simulink model "TV_2017old"  (R2016a)
settings: Solver=FixedStepAuto  StartTime=0.0  StopTime=inf  FixedStep=0.001  RelTol=1e-3
PreLoadFcn:
  | TV_2017_parameters
values from neighbouring files (symbols this model uses):
  battery_voltage = single(530)    [HIL_parameters.m]    (also in HIL_parameters_2018.m; TV_2017_parameters.m; TV_2017_parameters_VD.m)
  car_params = Simulink_Car_params    [HIL_parameters.m]    (also in HIL_parameters_2018.m; TV_2017_parameters.m; TV_2017_parameters_VD.m)
  i_Diff = 16    [HIL_parameters.m]    (also in HIL_parameters_2018.m; TV_2017_parameters.m)
  Kp = 1    [HIL_parameters.m]    (also in HIL_parameters_2018.m; TV_2017_parameters.m; TV_2017_parameters_VD.m)
  motor_data = struct    [HIL_parameters.m]    (also in HIL_parameters_2018.m; TV_2017_parameters.m)
  powerLimitControl = Simulink_el    [HIL_parameters.m]    (also in HIL_parameters_2018.m; TV_2017_parameters.m; TV_2017_parameters_VD.m)
  settings = Simulink_Settings    [HIL_parameters.m]    (also in HIL_parameters_2018.m; TV_2017_parameters.m; TV_2017_parameters_VD.m)
  SpdC_BCC = 0    [HIL_parameters.m]    (also in HIL_parameters_2018.m; TV_2017_parameters.m; TV_2017_parameters_VD.m)
  Speed_Neg_sat = -21    [HIL_parameters.m]    (also in HIL_parameters_2018.m; TV_2017_parameters.m; TV_2017_parameters_VD.m)
  Speed_Pos_sat = 21    [HIL_parameters.m]    (also in HIL_parameters_2018.m; TV_2017_parameters.m; TV_2017_parameters_VD.m)
  SteeringAngleFL = [-23.80 -22.65 -21.50 -20.34 -19.18 -18.03 -16.86 -15.70 -14.53 -13.35 -12.18 -10.99 -9.80 -8.61 -7.40 -6.19 -4.97 -3.75 -2.51 -1.26 0 1.27 2.56 3.85 5.17 6.50 7.84 9.21 10.59 12.00 13.42 14.88 16.36 17.87 19.41 20.99 22.61 24.26 25.97 27.73 29.54]    [CarSetupAnalysis2018.m]    (also in HIL_parameters_2018.m; TV_2017_parameters.m; TV_2017_parameters_VD.m = [-24.129 -22.950 -21.772 -20.593 -19.413 -18.232 -17.050 -15)
  SteeringAngleFR = [-29.54 -27.73 -25.97 -24.26 -22.61 -20.99 -19.41 -17.87 -16.36 -14.88 -13.42 -12.00 -10.59 -9.21 -7.84 -6.50 -5.17 -3.85 -2.56 -1.27 0 1.26 2.51 3.75 4.97 6.19 7.40 8.61 9.80 10.99 12.18 13.35 14.53 15.70 16.86 18.03 19.18 20.34 21.50 22.65 23.80]    [CarSetupAnalysis2018.m]    (also in HIL_parameters_2018.m; TV_2017_parameters.m; TV_2017_parameters_VD.m = [-29.3050 -27.5340 -25.8140 -24.1410 -22.5110 -20.9180 -19.3)
  SteeringWhAngle = [-105 -99.75 -94.5 -89.25 -84 -78.75 -73.5 -68.25 -63 -57.75 -52.5 -47.25 -42 -36.75 -31.5 -26.25 -21.0 -15.75 -10.5 -5.25 0.0 5.25 10.50 15.75 21.00 26.25 31.50 36.75 42.00 47.25 52.50 57.75  63.00 68.25 73.50 78.75 84.00 89.25 94.50 99.75 105.00]    [TV_2017_parameters_VD.m]
  Tn_n = 0    [HIL_parameters.m]    (also in HIL_parameters_2018.m; TV_2017_parameters.m; TV_2017_parameters_VD.m)
  tractionControl = Simulink_tc    [HIL_parameters.m]    (also in HIL_parameters_2018.m; IterativeTractionControlTuning.m; TV_2017_parameters.m; TV_2017_parameters_VD.m)
  yawRateControl = Simulink_yawRate    [HIL_parameters.m]    (also in HIL_parameters_2018.m; TV_2017_parameters.m; TV_2017_parameters_VD.m)
undefined symbols (not defined in the file or in its folder): DiscIntNeverNeededParam, magnitude, speedEstimation, TC_Decr_Gas, TC_Derivative, TC_Incr_Gas, TC_On, TC_Relay_Off, TC_Relay_On
libraries: CarMaker4SL x274, simulink_extras x45, simulink x37, dspfdesign x2
(part 8 of 14)

== matlab function TV_2017old/CarMaker/Estimations/EstimateVx/velocity_Estimation ==
  data: sensors input Bus: SensorInputs; V_est_x output; normalForces input Bus: normalForces; settings parameter; car_params parameter; speedEstimation parameter
function V_est_x  = velocityEstimation(sensors,normalForces,settings,car_params,speedEstimation)
%#codegen


persistent firstIteration;
persistent v;
persistent error;
persistent K;
persistent drift;

k_FL = single(0); % Gain 
k_FR = single(0); % Gain
k_RL = single(0); % Gain
k_RR = single(0); % Gain
% Gains for trusting, not trusting wheel speed measurements
Hg = speedEstimation.High_gain;
Lg = speedEstimation.Low_gain;
% Variances
all_Var = single(0); % Variance for all measurements
front_rear_Var = single(0);
front_Var = single(0);
rear_Var = single(0);
left_Var = single(0);
right_Var = single(0);
% LIMITS:
velocity_deviation_limit = speedEstimation.velocity_deviation_limit;
lim = speedEstimation.variance_limit;
RPM_derivative_limit = speedEstimation.RPM_derivative_limit;

% Measurement vector
C = [1;1;1;1]; % Create four copies of predicted vx


c = single(2*pi/(car_params.GR*60));

t = settings.control_system_sample_time;
%Weights taken from wikipedia
%sg_Weight = single( [ 1; -8; 0; 8; -1] );
sg_Weight = single( [ -1; 8; 0; -8; 1] );
%sg_Weight = single([0.3; 0.1; -0.1 ; -0.3]);
%sg_Weight = single([1; -1; 0 ; -0]);
% ------------------------------
% COPY VARIABLES EACH TIMESTEP
% ------------------------------
S = sensors.steering_wheel_angle; % Steering angle in rad( Mean of front wheels)
ax = sensors.ax; % Should be true linear acceleration compensated for roll angle
%Fz, used to determine what wheel speeds to trust.
Fz = [normalForces.FL, normalForces.FR, normalForces.RL ,normalForces.RR];
% Determine CoG Vx from motor RPM. Simple atm. Not considering vy.
Whl_v_FL = sensors.RPM_FL*c*car_params.r_eff*cos(S) + sensors.yawRate*car_params.t_f;
Whl_v_FR = sensors.RPM_FR*c*car_params.r_eff*cos(S) - sensors.yawRate*car_params.t_f;
Whl_v_RL = sensors.RPM_RL*c*car_params.r_eff + sensors.yawRate*car_params.t_r;
Whl_v_RR = sensors.RPM_RR*c*car_params.r_eff - sensors.yawRate*car_params.t_r;
whl_speed.v_FL = Whl_v_FL;
whl_speed.v_FR = Whl_v_FR;
whl_speed.v_RL = Whl_v_RL;
whl_speed.v_RR = Whl_v_RR;


RPM = [sensors.RPM_FL, sensors.RPM_FR, sensors.RPM_RL, sensors.RPM_RR]';
% Measurement vector, compensated RPMS
Y_meas = [Whl_v_FL, Whl_v_FR, Whl_v_RL, Whl_v_RR]';
% Input Derivative of RPM
rateRPM_FL = sensors.RPM_der_FL;
rateRPM_FR = sensors.RPM_der_FR;
rateRPM_RL = sensors.RPM_der_RL;
rateRPM_RR = sensors.RPM_der_RR;

% Different sums of normal forces, used to determine what wheels to trust
left_Fz = sum(Fz([1 3]));
right_Fz = sum(Fz([2 4]));
front_Fz = sum(Fz(1:2));
rear_Fz = sum(Fz(3:4));
% ALGORITHM
if (isempty(firstIteration))
    K = single(ones(1,4));
    v = single(0);
    V_est_x = v;
    error = Y_meas- C*v;
    firstIteration = 2;
    drift = single(0);
else
    v_ins = sensors.V_x_INS + 0.05 + drift;
    mean_WhlV = max(0.001,mean(Y_meas));
    mean_front_WhlV = max(0.001,mean(Y_meas(1:2)));
    mean_rear_WhlV  = max(0.001,mean(Y_meas(3:4)));
    mean_left_WhlV  = max(0.001,mean(Y_meas([1 3])));
    mean_right_WhlV = max(0.001,mean(Y_meas([2 4])));

    all_Var = var(Y_meas,1)/mean_WhlV;
    front_rear_Var = var([mean_front_WhlV, mean_rear_WhlV],1)/mean_WhlV;
    front_Var = var(Y_meas(1:2),1)/mean_front_WhlV;
    rear_Var  = var(Y_meas(3:4),1)/mean_rear_WhlV;
    
    left_Var    = var(Y_meas([1 3]),1)/mean_left_WhlV;
    right_Var   = var(Y_meas([2 4]),1)/mean_right_WhlV;   
    
    if ( (abs(Whl_v_FL - v_ins) > velocity_deviation_limit)...
       && (abs(Whl_v_FR - v_ins) > velocity_deviation_limit)...
       && (abs(Whl_v_RL - v_ins) > velocity_deviation_limit)...
       && (abs(Whl_v_RR - v_ins) > velocity_deviation_limit) )
        
        K = [Lg, Lg, Lg, Lg];
    elseif (all_Var  < lim ) 
        % low variance for all wheels.
        % Check derivative of motor RPM
        if ( (rateRPM_FL > RPM_derivative_limit) ||...
             (rateRPM_FR > RPM_derivative_limit) ||...
             (rateRPM_RL > RPM_derivative_limit) ||...
             (rateRPM_RR > RPM_derivative_limit))
            K = [Lg, Lg, Lg, Lg];
        % Rate of change of RPM can be low but slip rate is large
        % Check against drifting INS velocity 
        else
            K = [Hg, Hg ,Hg ,Hg];
        end
    % Variance is high. What wheel(s) are causing this.. 
    % STRUCTURE:
    % 1 = FRONT AND REAR DIFFER
    % 2 = LEFT AND RIGHT DIFFER
    % 3 = FL WRONG
    % 4 = FR WRONG
    % 5 = RL WRONG
    % 6 = RR WRONG
    % 7 Combinations of 3-6 that are not handled in 1-2.
    
    %1: FRONT AND REAR DIFFER
    elseif( (right_Var > front_Var) && (right_Var > rear_Var)...
            && (left_Var > front_Var) && (left_Var > rear_Var))
        % High variance between front and rear, and low variance 
        % at front and rear.
        
        % Also need to check if front/rear wheels are slippin    
        % Front wheels over limit while rear is ok
        if (((rateRPM_FL > RPM_derivative_limit) ||...
             (rateRPM_FR > RPM_derivative_limit)) &&...
            ((rateRPM_RL < RPM_derivative_limit) ||...
             (rateRPM_RR < RPM_derivative_limit)) )
             
            K = [Lg, Lg, Hg, Hg];
        % Rear wheels over limit while front is ok
        elseif ( ((rateRPM_FL < RPM_derivative_limit) ||...
                 (rateRPM_FR < RPM_derivative_limit)) &&...
                ((rateRPM_RL > RPM_derivative_limit) ||...
                 (rateRPM_RR > RPM_derivative_limit)) )
             K = [Hg, Hg, Lg, Lg];
        % All are over limit
        elseif  ((rateRPM_FL > RPM_derivative_limit) &&...
                 (rateRPM_FR > RPM_derivative_limit) &&...
                 (rateRPM_RL > RPM_derivative_limit) &&...
                 (rateRPM_RR > RPM_derivative_limit) ) 
              K = [Lg, Lg, Lg, Lg];
              
        % The rate of change of RPM will flatten out and the high
        % slip ratio will still exist. Handle this
        
        % Check big difference in wheel speeds
        % Two cases. Driving and braking. 
        
        % Driving. Need logic to determine driving/braking
        elseif ( (RPM(1) + RPM(2)) > (RPM(3) + RPM(4)) )
            K = [Lg, Lg, Hg, Hg];
        elseif ( (RPM(1) + RPM(2)) < (RPM(3) + RPM(4)) )
            K = [Hg, Hg, Lg, Lg];
            % If frontFZ - rearFZ < 0, then FL is set to 0
            % Else it is set to a positive gain
%             k_FL = (1/abs(front_Fz-rear_Fz))*max(0,front_Fz - rear_Fz);
%             k_FR = (1/abs(front_Fz-rear_Fz))*max(0,front_Fz - rear_Fz);
% 
%             k_RL = (1/abs(rear_Fz-front_Fz))*max(0,rear_Fz-front_Fz)*0.5;
%             k_RR = (1/abs(rear_Fz-front_Fz))*max(0,rear_Fz-front_Fz)*0.5;
%            K = [k_FL, k_FR, k_RL, k_RR];
        end
    %2: LEFT AND RIGHT WHEELS DIFFER
    elseif ( ((front_Var > right_Var) && (rear_Var > right_Var)) ||...
            ( (front_Var > left_Var) && (rear_Var > left_Var)))
   
        k_FL = (1/abs(left_Fz-right_Fz))*max(0,left_Fz - right_Fz);
        k_RL = (1/abs(left_Fz-right_Fz))*max(0,left_Fz - right_Fz);
        
        k_FR = (1/abs(right_Fz-left_Fz))*max(0,right_Fz-left_Fz);
        k_RR = (1/abs(right_Fz-left_Fz))*max(0,right_Fz-left_Fz);
        
        K = [k_FL, k_FR, k_RL, k_RR];
        
    %3: FL WRONG
    elseif ( (left_Var > rear_Var) && (left_Var > right_Var)...
            && (front_Var > rear_Var) )
        k_FL = single(0);
        k_FR = single(0);
        k_RL = single(1);
        k_RR = single(1);
        K = [k_FL, k_FR, k_RL, k_RR];
    %4: FR WRONG
    elseif ( (right_Var > rear_Var) && (right_Var > left_Var)...
            && (front_Var > rear_Var))
        k_FL = single(0);
        k_FR = single(0);
        k_RL = single(1);
        k_RR = single(1);
        K = [k_FL, k_FR, k_RL, k_RR]; 
    %5: RL WRONG
    elseif ( (left_Var > front_Var) && (left_Var > right_Var)...
            && (rear_Var > front_Var))
        
        k_FL = single(1);
        k_FR = single(1);
        k_RL = single(0);
        k_RR = single(0);
        K = [k_FL, k_FR, k_RL, k_RR]; 
        
    %5: RR WRONG    
    elseif ( (right_Var > front_Var) && (right_Var > left_Var)...
            && (rear_Var > front_Var))
        k_FL = single(1);
        k_FR = single(1);
        k_RL = single(0);
        k_RR = single(0);
        K = [k_FL, k_FR, k_RL, k_RR]; 
    else
        k_FL = single(0);
        k_FR = single(0);
        k_RL = single(0);
        k_RR = single(0);
        K = [k_FL, k_FR, k_RL, k_RR]; 
    end
    
    drift = drift + 0.03*t;
   
    %v = v + t*ax;
    v = v + t*(ax + K*error);
    error = Y_meas - C*v ;
    V_est_x = 0.98*v;
end
end

== matlab function TV_2017old/CarMaker/Control_System /Throttle // Brake Mapping ==
  data: states input; settings parameter; T_req output; car_params parameter
function T_req = pedalMapping(states,settings,car_params)
%#codegen

    KERS_pos = states.KERS_pos;
    throttle = min(1,states.Input_throttle);
    T_req = single(0);
    Fx_req = single(0);
    max_drive_torque = settings.max_motor_torque*4;
    max_brake_torque = settings.max_motor_brake_torque*4;
    
   persistent firstIteration;
   persistent KERS_allowed;
   
   % Hysteresis on KERS pedal input to avoid oscillation around 
   % allowed KERS speed. 
   if isempty(firstIteration)
      firstIteration = 2; %
      KERS_allowed = uint32(0);
   else
      % Hysteresis around the minimum KERS speed
       if     ( (KERS_allowed == 0) && (states.V_x > settings.KERS_speed_limit_hyst_high) )
           KERS_allowed = uint32(1);
       elseif ( (KERS_allowed == 1) && (states.V_x < settings.KERS_speed_limit_hyst_low) )
           KERS_allowed = uint32(0);
       end          
   end   
  if (settings.KERS_active == 1) 
      T_req = max_drive_torque*throttle  -  max_brake_torque*KERS_pos * single(KERS_allowed) ;
  else
      T_req = max_drive_torque*throttle ;
  end  
end

== matlab function TV_2017old/CarMaker/Estimations/Fz_Estimation_acceleration based/Fz_acc_est ==
  data: sensors input Bus: SensorInputs; Fz_acc_est output Bus: normalForces; car_params parameter; alfa_r_acc output
function [Fz_acc_est, alfa_r_acc] =  FzEstAcc(sensors , car_params)
%#codegen
g = 9.81;
ax = sensors.ax;
ay = sensors.ay;

total_mass = 245;
sprung_mass = 124+70;
unsprung_front = car_params.unsprung_mass_per_wheel_newton_front;
unspring_rear = car_params.unsprung_mass_per_wheel_newton_rear;
cg_z = 0.300;%car_params.CoG_height;
t_f = car_params.t_f;
t_r = car_params.t_r;
l_f = car_params.l_f;%Distance CoG to front axle
l_r = car_params.l_r;%Distance CoG to rear axle

K_ax = 1.25;
K_ay = 1.20;

%estimate forces from spring, damper and ARB
Fz_acc_est.FL = g*sprung_mass*0.25 + unsprung_front - K_ax*0.25*ax*sprung_mass*cg_z/l_f - K_ay*0.25*ay*sprung_mass*cg_z/t_f;
Fz_acc_est.FR = g*sprung_mass*0.25 + unsprung_front - K_ax*0.25*ax*sprung_mass*cg_z/l_f + K_ay*0.25*ay*sprung_mass*cg_z/t_f;
Fz_acc_est.RL = g*sprung_mass*0.25 + unspring_rear  + K_ax*0.25*ax*sprung_mass*cg_z/l_r - K_ay*0.25*ay*sprung_mass*cg_z/t_r;
Fz_acc_est.RR = g*sprung_mass*0.25 + unspring_rear  + K_ax*0.25*ax*sprung_mass*cg_z/l_r + K_ay*0.25*ay*sprung_mass*cg_z/t_r;

alfa_r_acc = (1.5+ax/g)/(3);

== matlab function TV_2017old/CarMaker/Estimations/SR_Calculation/Slip ratio ==
  data: V_x input; SR output Bus: SR; whl_v input Bus: Whl_speed; sensor input; car_params parameter
function SR = slipRatioCalculation(V_x,whl_v,sensor,car_params)
%#codegen

vx_to_wheel_factor = single(0.6);
vx_omega = sensor.yawRate*vx_to_wheel_factor;

Vx_FL = -vx_omega + V_x;
Vx_FR =  vx_omega + V_x;
Vx_RL = -vx_omega + V_x;
Vx_RR =  vx_omega + V_x;


SR.FL = single((whl_v.FL - Vx_FL) / max([1, abs(Vx_FL)]));    
SR.FR = single((whl_v.FR - Vx_FR) / max([1, abs(Vx_FR)]));
SR.RL = single((whl_v.RL - Vx_RL) / max([1, abs(Vx_RL)]));
SR.RR = single((whl_v.RR - Vx_RR) / max([1, abs(Vx_RR)]));

end

== matlab function TV_2017old/CarMaker/Estimations/RPM_to_linearVelocity/whl_v_calculation ==
  data: sensors input Bus: SensorInputs; meanWheelAngle input; car_params parameter; whl_speed output Bus: Whl_speed
function whl_speed = rpmToWhlVelocity(sensors,meanWheelAngle,car_params)
%#codegen

S = meanWheelAngle; % Steering angle in rad( Mean of front wheels)
c = single(2*pi/(car_params.GR*60));

% Determine CoG Vx from motor RPM. Simple atm. Not considering vy.
whl_speed.FL = sensors.RPM_FL*c*car_params.r_eff*cos(S) ;%+ sensors.yawRate*car_params.t_f;
whl_speed.FR = sensors.RPM_FR*c*car_params.r_eff*cos(S) ;%- sensors.yawRate*car_params.t_f;
whl_speed.RL = sensors.RPM_RL*c*car_params.r_eff        ;%+ sensors.yawRate*car_params.t_r;
whl_speed.RR = sensors.RPM_RR*c*car_params.r_eff        ;%- sensors.yawRate*car_params.t_r;

== matlab function TV_2017old/CarMaker/Estimations/Fx_Estimation/EstimateFx ==
  data: car_params parameter; Fx output Bus: Fx; sensors input Bus: SensorInputs; T_motor output Bus: T_motor
function [Fx, T_motor] = estimateFx(car_params, sensors)
%#codegen
Iq_FL = sensors.Iq_FL;
Iq_FR = sensors.Iq_FR;
Iq_RL = sensors.Iq_RL;
Iq_RR = sensors.Iq_RR;

Id_FL = sensors.Id_FL;
Id_FR = sensors.Id_FR;
Id_RL = sensors.Id_RL;
Id_RR = sensors.Id_RR;

Kt = car_params.Kt;     % Torque constant
Lq = car_params.Lq;     % Quadrature axis inductance 
Ld = car_params.Ld;     % Direct access inductance
Jw = car_params.Jw;     % Motor inertia
R  = car_params.r_eff;  % Radius center of rim to tire contact
GR = car_params.GR;     % Gear ratio
% Convert RPM Derivative to angular acceleration
c = single(2*pi/(GR*60));
ang_acc_FL = c*sensors.RPM_der_FL;
ang_acc_FR = c*sensors.RPM_der_FR;
ang_acc_RL = c*sensors.RPM_der_RL;
ang_acc_RR = c*sensors.RPM_der_RR;

% T_motor.FL = (Iq_FL*Kt*sqrt(2)-(Lq-Ld)*Id_FL);
% T_motor.FR = (Iq_FR*Kt*sqrt(2)-(Lq-Ld)*Id_FR);
% T_motor.RL = (Iq_RL*Kt*sqrt(2)-(Lq-Ld)*Id_RL);
% T_motor.RR = (Iq_RR*Kt*sqrt(2)-(Lq-Ld)*Id_RR);

T_motor.FL = (Iq_FL*Kt);
T_motor.FR = (Iq_FR*Kt);
T_motor.RL = (Iq_RL*Kt);
T_motor.RR = (Iq_RR*Kt);
%T_FL = T_CM.FL;
%T_FR = T_CM.FR;
%T_RL = T_CM.RL;
%T_RR = T_CM.RR;


Fx.FL = (T_motor.FL*GR - Jw*ang_acc_FL)/R;
Fx.FR = (T_motor.FR*GR - Jw*ang_acc_FR)/R;
Fx.RL = (T_motor.RL*GR - Jw*ang_acc_RL)/R;
Fx.RR = (T_motor.RR*GR - Jw*ang_acc_RR)/R;

== matlab function TV_2017old/CarMaker/Estimations/friction_estimation/estimateFrictionCoefficient ==
  data: Fx input Bus: Fx; mu output; mu_estimate output; Fz input Bus: normalForces; SR input Bus: SR; settings parameter; normLongTireForce output Bus: normLongTireForce
function [mu, mu_estimate, normLongTireForce]= estimateFrictionCoefficient(Fx,Fz,SR,settings)
%#codegen
persistent mu_FL;
persistent mu_FR;
persistent mu_RL;
persistent mu_RR;
persistent firstIteration;

mu_forget_factor = 0.001;  %kan legges in som parameter etter hvert. (Emil.17.10.2017)
mu_growth_factor = 0.0001;
mu_shrink_factor = 0.0001;
mu_full_slip_lim = 0.23;
mu_hi_slip_lim   = 0.13;
mu_lo_slip_lim   = 0.09;
mu_no_slip_lim   = 0.05;


if isempty(firstIteration)
    firstIteration = 2; %
    mu_FL = settings.mu;
    mu_FR = settings.mu;
    mu_RL = settings.mu;
    mu_RR = settings.mu;
    normLongTireForce.FL = single(0);
    normLongTireForce.FR = single(0);
    normLongTireForce.RL = single(0);
    normLongTireForce.RR = single(0);
   
      
else
    normLongTireForce.FL = (Fx.FL/Fz.FL);
    normLongTireForce.FR = (Fx.FR/Fz.FR);
    normLongTireForce.RL = (Fx.RL/Fz.RL);
    normLongTireForce.RR = (Fx.RR/Fz.RR);

%     %Front left
%     if (SR.FL > mu_lo_slip_lim) && (SR.FL < mu_hi_slip_lim)
%         mu_FL = (1-mu_forget_factor)*mu_FL + mu_forget_factor*normLongTireForce.FL;
%     elseif (SR.FL > mu_no_slip_lim) && (SR.FL < mu_lo_slip_lim)
%         mu_FL = (1-mu_forget_factor)*mu_FL + mu_growth_factor;
%     elseif (SR.FL > mu_lo_slip_lim) && (SR.FL < mu_full_slip_lim)
%         mu_FL = (1-mu_forget_factor)*mu_FL - mu_shrink_factor;        
%     end
%     %Front right
%     if (SR.FR > mu_lo_slip_lim) && (SR.FR < mu_hi_slip_lim)
%         mu_FR = (1-mu_forget_factor)*mu_FR + mu_forget_factor*normLongTireForce.FR;
%     elseif (SR.FR > mu_no_slip_lim) && (SR.FR < mu_lo_slip_lim)
%         mu_FR = (1-mu_forget_factor)*mu_FR + mu_growth_factor;
%     elseif (SR.FR > mu_lo_slip_lim) && (SR.FR < mu_full_slip_lim)
%         mu_FR = (1-mu_forget_factor)*mu_FR - mu_shrink_factor;        
%     end
%     %Rear left
%     if ( SR.RL > mu_lo_slip_lim) && (SR.RL < mu_hi_slip_lim)
%         mu_RL = (1-mu_forget_factor)*mu_RL + mu_forget_factor*normLongTireForce.RL;
%     elseif (SR.RL > mu_no_slip_lim) && (SR.RL < mu_lo_slip_lim)
%         mu_RL = (1-mu_forget_factor)*mu_RL + mu_growth_factor;
%     elseif (SR.RL > mu_lo_slip_lim) && (SR.RL < mu_full_slip_lim)
%         mu_RL = (1-mu_forget_factor)*mu_RL - mu_shrink_factor;        
%     end
%     %Rear right
%     if (SR.RR > mu_lo_slip_lim) && (SR.RR < mu_hi_slip_lim)
%        mu_RR = (1-mu_forget_factor)*mu_RR + mu_forget_factor*normLongTireForce.RR;
%     elseif (SR.RR > mu_no_slip_lim) && (SR.RR < mu_lo_slip_lim)
%        mu_RR = (1-mu_forget_factor)*mu_RR + mu_growth_factor;
%     elseif (SR.RR > mu_lo_slip_lim) && (SR.RR < mu_full_slip_lim)
%        mu_RR = (1-mu_forget_factor)*mu_RR - mu_shrink_factor;        
%     end
%}
end

mu = settings.mu;
mu_estimate = 0.25*(mu_FL+mu_FR+mu_RL+mu_RR);

end

== matlab function TV_2017old/CarMaker/Estimations/Fz_Estimation/1st_deriv/Diff_Function ==
  data: y_old output; y_old input; sig input; y output; delta_t input
function [y_old,y] = innerFunction(y_old, sig, delta_t)

y_old = circshift(y_old,1);
y_old(1) = sig;
        
M = length(y_old);
N = 3;
nu = 1;
j = 1;

k = 1:M;

x = phi(M,N,nu,j,k,delta_t) .* y_old;

y = sum(x);

end

function p = phi(M,N,nu,j,k,delta_t)

fac = (factorial(N + j + nu + 1) .*...
    factorial(N + 1)) ./...
    (M .* delta_t) .^ j;

[i,k2,k1,k] = ndgrid(0:nu + N,0:j,0:N-j,k);

eliminator = i > nu + k1 + k2;

evalIn = inPhi(M,N,nu,j,k,i,k1,k2);
evalIn(eliminator) = 0;

p = fac * sum(sum(sum(evalIn)));

p = p(:);

end

function p = inPhi(M,N,nu,j,k,i,k1,k2)

p = ((-1).^(N + i - k1 - k2) .*...
    ((k./M).^(N + i - k1 - k2 + 1) - ...
    ((k-1)./M).^(N + i - k1 - k2 + 1)))./...
    (factorial(k1) .* factorial(k2) .* factorial(i).*...
    factorial(N - j - k1) .*...
    factorial(j - k2) .*...
    factorial(N - k1 - k2) .*...
    factorial(nu - i + k1 + k2) .*...
    (N - k1 + 1) .*...
    (N + i -k1 - k2 + 1));

end

function n = factorial(n)

fac = [1;1;2;6;24;120;720;5040;40320;362880;3628800;39916800;479001600;6227020800.00000;87178291200.0000;1307674368000.00;20922789888000.0;355687428096000;6.40237370572800e+15;1.21645100408832e+17;2.43290200817664e+18;5.10909421717094e+19;1.12400072777761e+21;2.58520167388850e+22;6.20448401733239e+23;1.55112100433310e+25;4.03291461126606e+26;1.08888694504184e+28;3.04888344611714e+29;8.84176199373970e+30;2.65252859812191e+32;8.22283865417792e+33;2.63130836933694e+35;8.68331761881189e+36;2.95232799039604e+38;1.03331479663861e+40;3.71993326789901e+41;1.37637530912263e+43;5.23022617466601e+44;2.03978820811974e+46;8.15915283247898e+47;3.34525266131638e+49;1.40500611775288e+51;6.04152630633738e+52;2.65827157478845e+54;1.19622220865480e+56;5.50262215981209e+57;2.58623241511168e+59;1.24139155925361e+61;6.08281864034268e+62;3.04140932017134e+64];
n(n<0) = 0;
n = fac(n + 1);

end

== matlab function TV_2017old/CarMaker/Estimations/Fz_Estimation/2nd_deriv/Diff_Function ==
  data: y_old output; y_old input; sig input; y output; delta_t input
function [y_old,y] = innerFunction(y_old, sig, delta_t)

y_old = circshift(y_old,1);
y_old(1) = sig;
        
M = length(y_old);
N = 3;
nu = 0;
j = 2;

k = 1:M;

x = phi(M,N,nu,j,k,delta_t) .* y_old;

y = sum(x);

end

function p = phi(M,N,nu,j,k,delta_t)

fac = (factorial(N + j + nu + 1) .*...
    factorial(N + 1)) ./...
    (M .* delta_t) .^ j;

[i,k2,k1,k] = ndgrid(0:nu + N,0:j,0:N-j,k);

eliminator = i > nu + k1 + k2;

evalIn = inPhi(M,N,nu,j,k,i,k1,k2);
evalIn(eliminator) = 0;

p = fac * sum(sum(sum(evalIn)));

p = p(:);

end

function p = inPhi(M,N,nu,j,k,i,k1,k2)

p = ((-1).^(N + i - k1 - k2) .*...
    ((k./M).^(N + i - k1 - k2 + 1) - ...
    ((k-1)./M).^(N + i - k1 - k2 + 1)))./...
    (factorial(k1) .* factorial(k2) .* factorial(i).*...
    factorial(N - j - k1) .*...
    factorial(j - k2) .*...
    factorial(N - k1 - k2) .*...
    factorial(nu - i + k1 + k2) .*...
    (N - k1 + 1) .*...
    (N + i -k1 - k2 + 1));

end

function n = factorial(n)

fac = [1;1;2;6;24;120;720;5040;40320;362880;3628800;39916800;479001600;6227020800.00000;87178291200.0000;1307674368000.00;20922789888000.0;355687428096000;6.40237370572800e+15;1.21645100408832e+17;2.43290200817664e+18;5.10909421717094e+19;1.12400072777761e+21;2.58520167388850e+22;6.20448401733239e+23;1.55112100433310e+25;4.03291461126606e+26;1.08888694504184e+28;3.04888344611714e+29;8.84176199373970e+30;2.65252859812191e+32;8.22283865417792e+33;2.63130836933694e+35;8.68331761881189e+36;2.95232799039604e+38;1.03331479663861e+40;3.71993326789901e+41;1.37637530912263e+43;5.23022617466601e+44;2.03978820811974e+46;8.15915283247898e+47;3.34525266131638e+49;1.40500611775288e+51;6.04152630633738e+52;2.65827157478845e+54;1.19622220865480e+56;5.50262215981209e+57;2.58623241511168e+59;1.24139155925361e+61;6.08281864034268e+62;3.04140932017134e+64];
n(n<0) = 0;
n = fac(n + 1);

end

== matlab function TV_2017old/CarMaker/Control_System /Slip Rate Control /Traction Controllers/MATLAB Function ==
  data: Ti_FL input; Ti_FR input; Ti_lim output Bus: Ti_lim; Ti_RL input; Ti_RR input; TC_FL input; TC_FR input; TC_RL input; TC_RR input; states input Bus: States; T_req input
function Ti_lim =  TCOutputHandling(Ti_FL, Ti_FR, Ti_RL, Ti_RR, TC_FL,TC_FR,TC_RL,TC_RR,states, T_req)
%#codegen


Ti_lim.FL = Ti_FL + TC_FL;
Ti_lim.FR = Ti_FR + TC_FR;
Ti_lim.RL = Ti_RL + TC_RL;
Ti_lim.RR = Ti_RR + TC_RR;


% yawRate_p_lim = 0.3;
% ay_p_lim = 3;
% 
% straightline = uint32(0);
% 
% if ( (states.r > -yawRate_p_lim) && (states.r < yawRate_p_lim) &&...
%      (states.ay > -ay_p_lim) && (states.ay < ay_p_lim) )
%     straightline = 1;
% else
%     straightline = 0;
% end
% 
% 
% % FRONT SIDE
% n_cmp = single(-0.03);
% p_cmp = single(0.03);
% 
% % If driving ~ straightline then couple the outputs
% % Else, each TC works individually. 
% if      ( (straightline == 1) && (T_req > p_cmp) )
%     % Couple TC outputs to maintain stability on mu split surfaces 
%     % under acceleration and deceleration
%     Ti_lim.FL = max(0, (Ti_FL + min(TC_FL,TC_FR)));
%     Ti_lim.FR = max(0, (Ti_FR + min(TC_FL,TC_FR)));  
%     
%     Ti_lim.RL = max(0, (Ti_RL + min(TC_RL,TC_RR)));
%     Ti_lim.RR = max(0, (Ti_RR + min(TC_RL,TC_RR)));
%  
% elseif  ( (straightline == 1) && (T_req < n_cmp) )
%     % Couple TC outputs to maintain stability on mu split surfaces 
%     % under acceleration and deceleration
%     Ti_lim.FL = min(0, (Ti_FL + max(TC_FL,TC_FR) ) );   
%     Ti_lim.FR = min(0, (Ti_FR + max(TC_FL,TC_FR) ) );    
%     Ti_lim.RL = min(0, (Ti_RL + max(TC_RL,TC_RR) ) );
%     Ti_lim.RR = min(0, (Ti_RR + max(TC_RL,TC_RR) ) );   
% else
%     % Decouple TC outputs to avoid interferring too much with the stability
%     % of the vehicle while cornering. This is the DYC systems job. 
%     Ti_lim.FL = Ti_FL + TC_FL;
%     Ti_lim.FR = Ti_FR + TC_FR;
%     Ti_lim.RL = Ti_RL + TC_RL;
%     Ti_lim.RR = Ti_RR + TC_RR;
% end

end

== matlab function TV_2017old/CarMaker/Control_System /Slip Rate Control /SMC Traction Control/MATLAB Function ==
  data: Ti_FL input; Ti_FR input; Ti_lim output Bus: Ti_lim; Ti_RL input; Ti_RR input; TC_FL input; TC_FR input; TC_RL input; TC_RR input; states input Bus: States; T_req input
function Ti_lim =  TCOutputHandling(Ti_FL, Ti_FR, Ti_RL, Ti_RR, TC_FL,TC_FR,TC_RL,TC_RR,states, T_req)
%#codegen

yawRate_p_lim = 0.2;
ay_p_lim = 3;

straightline = uint32(0);

if ( (states.r > -yawRate_p_lim) && (states.r < yawRate_p_lim) && ...
     (states.ay > -ay_p_lim) && (states.ay < ay_p_lim) )
    straightline = 1;
else
    straightline = 0;
end


% Proposal : TC only active if yaw rate within some set

% FRONT SIDE
n_cmp = single(-0.03);
p_cmp = single(0.03);

% If driving ~ straightline then couple the outputs
% Else, each TC works individually. 
if      ( (straightline == 1) && (T_req > p_cmp) )
    % Couple TC outputs to maintain stability on mu split surfaces 
    % under acceleration and deceleration
    Ti_lim.FL = max(0, (Ti_FL + min(TC_FL,TC_FR) ) );
    Ti_lim.FR = max(0, (Ti_FR + min(TC_FL,TC_FR) ) );
    
    Ti_lim.RL = max(0, (Ti_RL + min(TC_RL,TC_RR) ) );
    Ti_lim.RR = max(0, (Ti_RR + min(TC_RL,TC_RR) ) );
 
elseif  ( (straightline) && (T_req < n_cmp) )
    % Couple TC outputs to maintain stability on mu split surfaces 
    % under acceleration and deceleration
    Ti_lim.FL = min(0, (Ti_FL + max(TC_FL,TC_FR) ) );
    Ti_lim.FR = min(0, (Ti_FR + max(TC_FL,TC_FR) ) );
    
    Ti_lim.RL = min(0, (Ti_RL + max(TC_RL,TC_RR) ) );
    Ti_lim.RR = min(0, (Ti_RR + max(TC_RL,TC_RR) ) );   
else
    % Decouple TC outputs to avoid interferring too much with the stability
    % of the vehicle while cornering. This is the DYC systems job. 
    Ti_lim.FL = Ti_FL + TC_FL;
    Ti_lim.FR = Ti_FR + TC_FR;
    Ti_lim.RL = Ti_RL + TC_RL;
    Ti_lim.RR = Ti_RR + TC_RR;
end

end




% if      ( (TC_FL < n_cmp) && (TC_FR < n_cmp) )
%     % add the most negative
% elseif  ( (TC_FL > p_cmp) && (TC_FR > p_cmp) )
%     % Add the most positive
%     
% elseif  ( (TC_FL < n_cmp) && (TC_FR > p_cmp) )
%     % Individual control
% elseif  ( (TC_FL > p_cmp) && (TC_FR < n_cmp) )
%     % Individual control
%     
%     
% elseif  ( (TC_FL > p_cmp) && (TC_FR < p_cmp) && (TC_FR > n_cmp) && (T_req < n_cmp) )
%     % One wants to add, other is fine and T_req < 0 which means it must be
%     % braking either straight or into a corner.. Add to both wheels, but do
%     % not exceed 0 torque.
%     
% elseif  ( (TC_FL < p_cmp) && (TC_FL > n_cmp) && (TC_FR > p_cmp)  && (T_req < n_cmp) )
%     % One wants to add, other is fine and T_req < 0 which means it must be
%     % braking either straight or into a corner.. Add to both wheels, but do
%     % not exceed 0 torque.    
%     
% elseif  ( (TC_FL < n_cmp) && ( (TC_FR < p_cmp) && (TC_FR > n_cmp) ) ...
%           && (T_req > p_cmp) && (straightline))
%     % One wants to subtract, other is fine and T_req > 0 and straightline
%     % which means mu split acceleration.
%     
%  elseif  ( (TC_FL > n_cmp) && (TC_FL < p_cmp) && (TC_FR < n_cmp) ) ...
%           && (T_req > p_cmp) && (straightline))
%     % One wants to subtract, other is fine and T_req > 0 and straightline
%     % which means mu split acceleration.    
%     
% elseif  ( (TC_FL < n_cmp) &&  (TC_FR < p_cmp) && (TC_FR > n_cmp) ...
%            && (not(straightline)))
%     % One wants to subtract, other is fine and T_req > 0 and straightline
%     % is false which means
%     
%  elseif  ( (TC_FL > n_cmp) && (TC_FL < p_cmp) && (TC_FR < n_cmp)  ...
%            && (not(straightline)))
%     % One wants to subtract, other is fine and T_req > 0 and straightline
%     % which means mu split acceleration.       
% elseif  
%     
%     
% y = u;

== matlab function TV_2017old/CarMaker/Control_System /Slip Rate Control /SMC Traction Control/MATLAB Function1 ==
  data: states input Bus: States; SR_FL output; SR_FR output; SR_RL output; SR_RR output; vx output
function [SR_FL,SR_FR,SR_RL,SR_RR,vx] = extractSlipRatios(states)
%#codegen


SR_FL = states.SR_FL;
SR_FR = states.SR_FR;
SR_RL = states.SR_RL;
SR_RR = states.SR_RR;

vx = states.V_x;

== matlab function TV_2017old/CarMaker/Control_System /Power Limit Torque Reduction Controller /Motorestimates/extractPower2 ==
  data: T_FL output; states input; RPM_FL output; T_FR output; RPM_FR output; T_RL output; RPM_RL output; T_RR output; RPM_RR output; Ti_lim input
function [T_FL, RPM_FL, T_FR, RPM_FR, T_RL, RPM_RL, T_RR, RPM_RR]= extractRPM(states, Ti_lim)
%#codegen
RPM_FL = states.RPM_FL;
RPM_FR = states.RPM_FR;
RPM_RL = states.RPM_RL;
RPM_RR = states.RPM_RR;

T_FL = Ti_lim.FL;
T_FR = Ti_lim.FR;
T_RL = Ti_lim.RL;
T_RR = Ti_lim.RR;

end

== matlab function TV_2017old/CarMaker/Control_System /Slip Rate Control /SMC Traction Control/Slip Rate FL/SMC ==
  data: muOfSlip input; TC output; SR input; SR_ref input; car_params parameter; states input; K input
function TC = fcn(muOfSlip,SR,SR_ref,car_params, states,K)
%#codegen
Jr = 0.2;
GR = car_params.GR;
r = car_params.r_eff;
m = car_params.mass;
Fz_FL = states.Fz_FL;
%slip = ((Jr/(m*r^2*(1-SR))) +1 )*muOfSlip*Fz_FL*r

ySlip = (r*(1-SR)^2)/(Jr*states.V_x);
force = muOfSlip*Fz_FL*r/GR
TC = force - (K/(ySlip))*sign(SR-SR_ref)*min(1,abs(SR-SR_ref));

== matlab function TV_2017old/CarMaker/Control_System /Slip Rate Control /SMC Traction Control/Slip Rate FL1/SMC ==
  data: muOfSlip input; TC output; SR input; SR_ref input; car_params parameter; states input; K input
function TC = fcn(muOfSlip,SR,SR_ref,car_params, states,K)
%#codegen
Jr = 0.2;
GR = car_params.GR;
r = car_params.r_eff;
m = car_params.mass;
Fz_FR = states.Fz_FR;
%slip = ((Jr/(m*r^2*(1-SR))) +1 )*muOfSlip*Fz_FL*r
ySlip = (r*(1-SR)^2)/(Jr*states.V_x);
force = muOfSlip*Fz_FR*r/GR
TC = force - (K/(ySlip))*sign(SR-SR_ref)*min(1,abs(SR-SR_ref));

== matlab function TV_2017old/CarMaker/Control_System /Slip Rate Control /SMC Traction Control/Slip Rate FL2/SMC ==
  data: muOfSlip input; TC output; SR input; SR_ref input; car_params parameter; states input; K input
function TC = fcn(muOfSlip,SR,SR_ref,car_params, states,K)
%#codegen
Jr = 0.2;
GR = car_params.GR;
r = car_params.r_eff;
m = car_params.mass;
Fz_RL = states.Fz_RL;
%slip = ((Jr/(m*r^2*(1-SR))) +1 )*muOfSlip*Fz_FL*r
ySlip = (r*(1-SR)^2)/(Jr*states.V_x);
force = muOfSlip*Fz_RL*r/GR
TC = force - (K/(ySlip))*sign(SR-SR_ref)*min(1,abs(SR-SR_ref));

== matlab function TV_2017old/CarMaker/Control_System /Slip Rate Control /SMC Traction Control/Slip Rate FL3/SMC ==
  data: muOfSlip input; TC output; SR input; SR_ref input; car_params parameter; states input; K input
function TC = fcn(muOfSlip,SR,SR_ref,car_params, states,K)
%#codegen
Jr = 0.2;
GR = car_params.GR;
r = car_params.r_eff;
m = car_params.mass;
Fz_RR = states.Fz_RR;
%slip = ((Jr/(m*r^2*(1-SR))) +1 )*muOfSlip*Fz_FL*r
ySlip = (r*(1-SR)^2)/(Jr*states.V_x);
force = muOfSlip*Fz_RR*r/GR
TC = force - (K/(ySlip))*sign(SR-SR_ref)*min(1,abs(SR-SR_ref));

== matlab function TV_2017old/CarMaker/Estimations/calculateMeanWheelAngle/calculateWheelangleandSpeed ==
  data: mean_wheel_angle output single; sensor input Bus: SensorInputs; mean_wheel_speed output single
function [mean_wheel_angle, mean_wheel_speed] = calculateWheelAngle(sensor)
%#codegen

% Right now assumes rad for angle, and rad/s for speed
mean_wheel_angle    = single(0.2536*sensor.steering_wheel_angle);
mean_wheel_speed    = single(0.2536*sensor.steering_wheel_speed);

end

== matlab function TV_2017old/CarMaker/Estimations/Fz_Estimation/FzEstDamper ==
  data: sensors input Bus: SensorInputs; Fz_damp_FL input; Fz_damp_FR input; Fz_damper_est output Bus: normalForces; Fz_damp_RL input; Fz_damp_RR input; car_params parameter; alfa_r output
function [Fz_damper_est, alfa_r] =  FzEstDamp(sensors, Fz_damp_FL, Fz_damp_FR, Fz_damp_RL, Fz_damp_RR, car_params)
%#codegen

Ks_front    = car_params.spring_constant_front;
Ks_rear     = car_params.spring_constant_rear;
unsprung_front = car_params.unsprung_mass_per_wheel_newton_front; 
unsprung_rear  = car_params.unsprung_mass_per_wheel_newton_rear; 
half_track_front =  car_params.t_f;
half_track_rear  =  car_params.t_r;
arb_Ks_front     = car_params.arb_f_Nm_rad;
arb_Ks_rear      = car_params.arb_r_Nm_rad;
damper_pos_FL = sensors.damper_pos_FL ;
damper_pos_FR = sensors.damper_pos_FR ;
damper_pos_RL = sensors.damper_pos_RL ;
damper_pos_RR = sensors.damper_pos_RR ;

FL_preload = car_params.preload_front_mm * Ks_front;% * 0.001;
FR_preload = car_params.preload_front_mm * Ks_front;% * 0.001;
RL_preload = car_params.preload_rear_mm * Ks_rear;% * 0.001;
RR_preload = car_params.preload_rear_mm * Ks_rear;% * 0.001;

%add unsprung mass to Fz estimate gradualy as spring compress (not during wheel lift )
add_unsprung_threshold = 2;
scale = 1 / add_unsprung_threshold;
FL_unsprung = single((unsprung_front+FL_preload) * scale *  max(   0,  min(    damper_pos_FL , single(add_unsprung_threshold)   )));
FR_unsprung = single((unsprung_front+FR_preload) * scale *  max(   0,  min(    damper_pos_FR , single(add_unsprung_threshold)   )));
RL_unsprung = single((unsprung_rear+RL_preload) * scale *  max(   0,  min(    damper_pos_RL , single(add_unsprung_threshold)   )));
RR_unsprung = single((unsprung_rear+RR_preload) * scale *  max(   0,  min(    damper_pos_RR , single(add_unsprung_threshold)   )));

%adjust estimate for ARB weight transfer

arb_transfer_f = arb_Ks_front * sensors.roll_angle * half_track_front; 
arb_transfer_r = arb_Ks_rear * sensors.roll_angle * half_track_rear; 
K_damp_front=800;
K_damp_rear =800;
%estimate forces from spring, damper and ARB
min_value = 200;
Fz_damper_est.FL = max(min_value ,  Ks_front*damper_pos_FL  + FL_unsprung);% - K_damp_front*Fz_damp_FL;%+ arb_transfer_f; % 
Fz_damper_est.FR = max(min_value ,  Ks_front*damper_pos_FR  + FR_unsprung);% - K_damp_front*Fz_damp_FR;%- arb_transfer_f; % 
Fz_damper_est.RL = max(min_value ,  Ks_rear*damper_pos_RL   + RL_unsprung);% - K_damp_rear*Fz_damp_RL;%+ arb_transfer_r; % 
Fz_damper_est.RR = max(min_value ,  Ks_rear*damper_pos_RR   + RR_unsprung);% - K_damp_rear*Fz_damp_RR;%- arb_transfer_r; % 

alfa_r = max(1,(Fz_damper_est.RL + Fz_damper_est.RR)) / max(1,(Fz_damper_est.FL + Fz_damper_est.FR + Fz_damper_est.RL + Fz_damper_est.RR));
